simulink subsystem "sub_signal"  (R2023b)
settings: Solver=VariableStepAuto  StartTime=0.0  StopTime=10.0  RelTol=1e-3
libraries: simulink x2
settings Model: Creator=ricfe  LastModifiedBy=ricfe

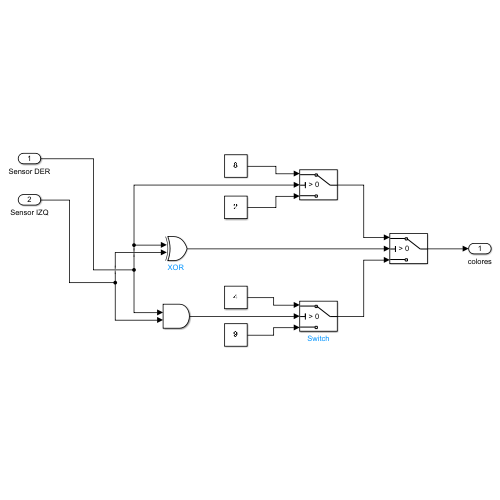
[thumbnail: Simulink's stored preview of the top-level diagram]
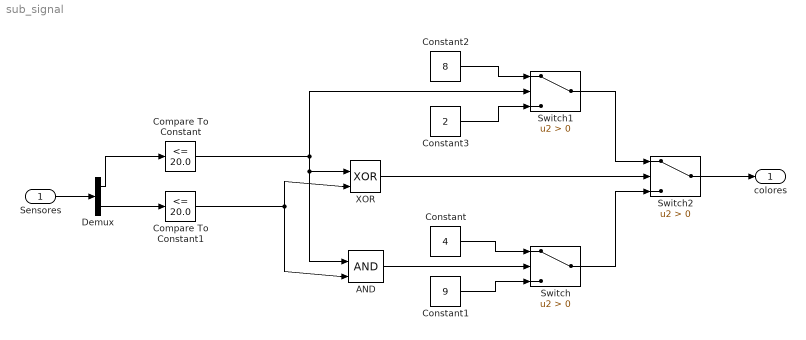
== system sub_signal ==
  Sensores : Inport
  AND : Logic  IconShape=distinctive  AllPortsSameDT=off  OutDataTypeStr=boolean
  Compare To Constant : simulink/Logic and Bit Operations/Compare To Constant  relop=<=  const=20.0  OutDataTypeStr=boolean
  Compare To Constant1 : simulink/Logic and Bit Operations/Compare To Constant  relop=<=  const=20.0  OutDataTypeStr=boolean
  Constant : Constant  Value=4
  Constant1 : Constant  Value=9
  Constant2 : Constant  Value=8
  Constant3 : Constant  Value=2
  Demux : Demux  Outputs=2
  Switch : Switch  Criteria=u2 > Threshold  SaturateOnIntegerOverflow=off  InputSameDT=off
  Switch1 : Switch  Criteria=u2 > Threshold  SaturateOnIntegerOverflow=off  InputSameDT=off
  Switch2 : Switch  Criteria=u2 > Threshold  SaturateOnIntegerOverflow=off  InputSameDT=off
  XOR : Logic  Operator=XOR  IconShape=distinctive  AllPortsSameDT=off  OutDataTypeStr=boolean
  colores : Outport
  wires:
  Demux/2 -> Compare To Constant1/1
  AND/1 -> Switch/2
  Constant/1 -> Switch/1
  Constant1/1 -> Switch/3
  Constant3/1 -> Switch1/3
  Constant2/1 -> Switch1/1
  XOR/1 -> Switch2/2
  Switch1/1 -> Switch2/1
  Switch/1 -> Switch2/3
  Switch2/1 -> colores/1
  Demux/1 -> Compare To Constant/1
  Sensores/1 -> Demux/1
  Compare To Constant/1 -> Switch1/2, XOR/1, AND/1
  Compare To Constant1/1 -> XOR/2, AND/2
